simulink model "l2_pj_experiment"  (Simulink 7.1)
settings: Solver=ode45  StartTime=0.0  StopTime=100  MaxStep=.1  RelTol=1e-3
model workspace (MAT data in the model file):
  b : Simulink.Parameter (value not decoded)
  Ts : Simulink.Parameter (value not decoded)
  plant_index : Simulink.Parameter (value not decoded)
  omega_traj : Simulink.Parameter (value not decoded)
  alpha : Simulink.Parameter (value not decoded)
  N : Simulink.Parameter (value not decoded)
  epsilon : Simulink.Parameter (value not decoded)
  kp : Simulink.Parameter (value not decoded)
  wp : Simulink.Parameter (value not decoded)
libraries: passive_control x9, simulink x5
settings Model: Creator=Administrator  LastModifiedBy=Administrator

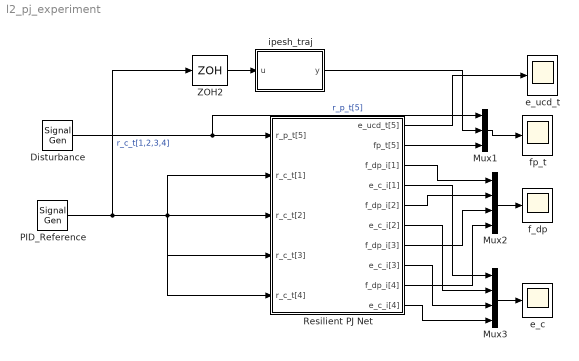
== system l2_pj_experiment ==
  Disturbance : SignalGenerator  WaveForm=square  Amplitude=.5  Frequency=.025
  Mux1 : Mux  Inputs=3
  Mux2 : Mux
  Mux3 : Mux
  PID_Reference : SignalGenerator  WaveForm=square  Frequency=.0125
  Resilient PJ Net : Subsystem
  ZOH2 : ZeroOrderHold  SampleTime=Ts
  e_c : Scope
      settings: SaveName=ScopeData2  SampleInput=on  SampleTime=Ts/10
  e_ucd_t : Scope
      settings: YMin=-1.1  YMax=1.1  SaveName=ScopeData3  SampleInput=on  SampleTime=Ts/10
  f_dp : Scope
      settings: TimeRange=100  SampleInput=on  SampleTime=Ts/10
  fp_t : Scope
      settings: TimeRange=100  YMin=-1.25  YMax=1.25  SampleInput=on  SampleTime=Ts/10
  ipesh_traj : Subsystem  mask{num=[omega_traj^2], den=[1,2*.9*omega_traj,omega_traj^2], Ts=Ts}
      mask prompts: num "H(s) num"; den "H(s) den"; Ts "Ts (sec)"
      mask init:
      | Hs=tf(num,den);
      | Hz=ipesh_transform(Hs,Ts);
  wires:
  PID_Reference/1 -> Resilient PJ Net/2(r_c_t[1]), Resilient PJ Net/3(r_c_t[2]), Resilient PJ Net/4(r_c_t[3]), Resilient PJ Net/5(r_c_t[4]), ZOH2/1  "r_c_t[1,2,3,4]"
  Disturbance/1 -> Resilient PJ Net/1(r_p_t[5]), Mux1/1  "r_p_t[5]"
  Mux2/1 -> f_dp/1
  Mux3/1 -> e_c/1
  Resilient PJ Net/1(e_ucd_t[5]) -> e_ucd_t/1
  Resilient PJ Net/10(e_c_i[4]) -> Mux3/4
  Resilient PJ Net/8(e_c_i[3]) -> Mux3/3
  Resilient PJ Net/6(e_c_i[2]) -> Mux3/2
  Resilient PJ Net/4(e_c_i[1]) -> Mux3/1
  Resilient PJ Net/3(f_dp_i[1]) -> Mux2/1
  Resilient PJ Net/5(f_dp_i[2]) -> Mux2/2
  Resilient PJ Net/7(f_dp_i[3]) -> Mux2/3
  Resilient PJ Net/9(f_dp_i[4]) -> Mux2/4
  Mux1/1 -> fp_t/1
  Resilient PJ Net/2(fp_t[5]) -> Mux1/3
  ZOH2/1 -> ipesh_traj/1(u)
  ipesh_traj/1(y) -> Mux1/2

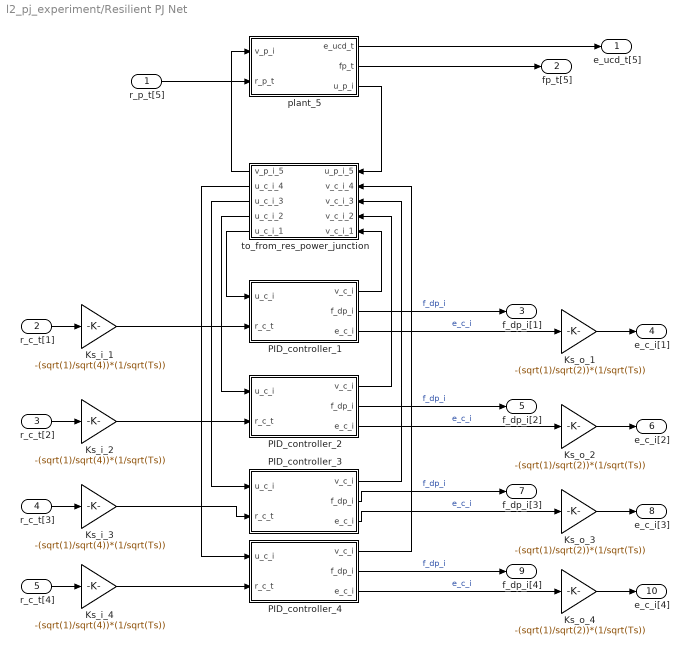
== system l2_pj_experiment/Resilient PJ Net ==
  r_p_t[5] : Inport
  r_c_t[1] : Inport  Port=2
  r_c_t[2] : Inport  Port=3
  r_c_t[3] : Inport  Port=4
  r_c_t[4] : Inport  Port=5
  Ks_i_{1..4} (4 alike) : Gain  Gain=-(sqrt(1)/sqrt(4))*(1/sqrt(Ts))  ParameterDataType=sfix(16)  ParameterScaling=2^0  OutDataType=sfix(16)  OutScaling=2^0
  Ks_o_{1..4} (4 alike) : Gain  Gain=-(sqrt(1)/sqrt(2))*(1/sqrt(Ts))  ParameterDataType=sfix(16)  ParameterScaling=2^0  OutDataType=sfix(16)  OutScaling=2^0
  PID_controller_1 : Subsystem
  PID_controller_2 : Subsystem
  PID_controller_3 : Subsystem
  PID_controller_4 : Subsystem
  plant_5 : Subsystem
  to_from_res_power_junction : Subsystem  Orientation=left
  e_ucd_t[5] : Outport
  fp_t[5] : Outport  Port=2
  f_dp_i[1] : Outport  Port=3
  e_c_i[1] : Outport  Port=4
  f_dp_i[2] : Outport  Port=5
  e_c_i[2] : Outport  Port=6
  f_dp_i[3] : Outport  Port=7
  e_c_i[3] : Outport  Port=8
  f_dp_i[4] : Outport  Port=9
  e_c_i[4] : Outport  Port=10
  wires:
  Ks_i_1/1 -> PID_controller_1/2(r_c_t)
  r_p_t[5]/1 -> plant_5/2(r_p_t)
  PID_controller_1/2(f_dp_i) -> f_dp_i[1]/1  "f_dp_i"
  r_c_t[1]/1 -> Ks_i_1/1
  PID_controller_1/3(e_c_i) -> Ks_o_1/1  "e_c_i"
  Ks_o_1/1 -> e_c_i[1]/1
  plant_5/1(e_ucd_t) -> e_ucd_t[5]/1
  plant_5/2(fp_t) -> fp_t[5]/1
  plant_5/3(u_p_i) -> to_from_res_power_junction/1(u_p_i_5)
  to_from_res_power_junction/1(v_p_i_5) -> plant_5/1(v_p_i)
  PID_controller_1/1(v_c_i) -> to_from_res_power_junction/5(v_c_i_1)
  to_from_res_power_junction/5(u_c_i_1) -> PID_controller_1/1(u_c_i)
  Ks_i_2/1 -> PID_controller_2/2(r_c_t)
  PID_controller_2/2(f_dp_i) -> f_dp_i[2]/1  "f_dp_i"
  r_c_t[2]/1 -> Ks_i_2/1
  PID_controller_2/3(e_c_i) -> Ks_o_2/1  "e_c_i"
  Ks_o_2/1 -> e_c_i[2]/1
  Ks_i_3/1 -> PID_controller_3/2(r_c_t)
  PID_controller_3/2(f_dp_i) -> f_dp_i[3]/1  "f_dp_i"
  r_c_t[3]/1 -> Ks_i_3/1
  PID_controller_3/3(e_c_i) -> Ks_o_3/1  "e_c_i"
  Ks_o_3/1 -> e_c_i[3]/1
  Ks_i_4/1 -> PID_controller_4/2(r_c_t)
  PID_controller_4/2(f_dp_i) -> f_dp_i[4]/1  "f_dp_i"
  r_c_t[4]/1 -> Ks_i_4/1
  PID_controller_4/3(e_c_i) -> Ks_o_4/1  "e_c_i"
  Ks_o_4/1 -> e_c_i[4]/1
  PID_controller_2/1(v_c_i) -> to_from_res_power_junction/4(v_c_i_2)
  to_from_res_power_junction/4(u_c_i_2) -> PID_controller_2/1(u_c_i)
  PID_controller_3/1(v_c_i) -> to_from_res_power_junction/3(v_c_i_3)
  to_from_res_power_junction/3(u_c_i_3) -> PID_controller_3/1(u_c_i)
  PID_controller_4/1(v_c_i) -> to_from_res_power_junction/2(v_c_i_4)
  to_from_res_power_junction/2(u_c_i_4) -> PID_controller_4/1(u_c_i)

== system l2_pj_experiment/ipesh_traj ==
  u : Inport
  ipesh : DiscreteTransferFcn  Numerator=Hz.num{1}  Denominator=Hz.den{1}  SampleTime=-1
  y : Outport
  wires:
  u/1 -> ipesh/1
  ipesh/1 -> y/1

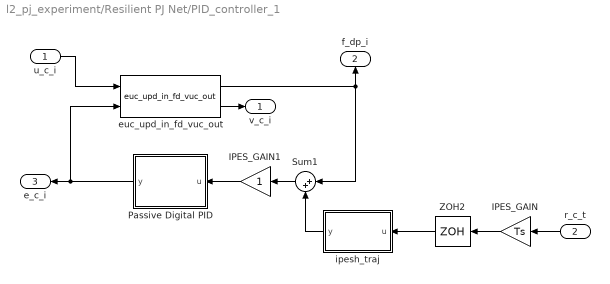
== system l2_pj_experiment/Resilient PJ Net/PID_controller_1 ==
  u_c_i : Inport
  r_c_t : Inport  Orientation=left  Port=2
  IPES_GAIN : Gain  Orientation=left  Gain=Ts  ParameterDataType=sfix(16)  ParameterScaling=2^0  OutDataType=sfix(16)  OutScaling=2^0
  IPES_GAIN1 : Gain  Orientation=left  ParameterDataType=sfix(16)  ParameterScaling=2^0  OutDataType=sfix(16)  OutScaling=2^0
  Passive Digital PID : Subsystem  Orientation=left  mask{kpk=kp, wpk=wp, alpha=alpha, N=N, Ts=Ts, epsilon=epsilon}
      mask prompts: kpk "Enter Plant Gains kpk (Vector)"; wpk "Enter Plant Frequencies wpk (Vector)"; alpha "Enter Alpha"; N "Enter N"; Ts "Sample Time [Ts] (seconds)"; epsilon "Enter epsiolon"
      mask init:
      | ksk=kpk./wpk;
      | kp=min(kpk);
      | wp=min(wpk);
      | wn=pi/Ts;
      | Kp=(1/3)*alpha*(wn+wp)/kp;
      | Ki=(1/3)*alpha*wn*(wn+wp)/kp;
      | Kd=(1/3)*alpha*(2/(N+1))*(wn+wp)/kp;
      | GIs=feedback(tf(Kp,[1,0]),epsilon);
      | GDs=Kd*tf([N*Ts/pi,1],[Ts/pi,1]);
  Sum1 : Sum  Orientation=left  Inputs=|++  OutDataType=sfix(16)  OutScaling=2^0
  ZOH2 : ZeroOrderHold  Orientation=left  SampleTime=Ts
  euc_upd_in_fd_vuc_out : passive_control/euc_upd_in_fd_vuc_out  SystemSampleTime=-1  b=b
  ipesh_traj : Subsystem  Orientation=left  mask{num=[omega_traj^2], den=[1,2*.9*omega_traj,omega_traj^2], Ts=Ts}
      mask prompts: num "H(s) num"; den "H(s) den"; Ts "Ts (sec)"
      mask init:
      | Hs=tf(num,den);
      | Hz=ipesh_transform(Hs,Ts);
  v_c_i : Outport
  f_dp_i : Outport  Orientation=up  Port=2
  e_c_i : Outport  Orientation=left  Port=3
  wires:
  euc_upd_in_fd_vuc_out/1 -> Sum1/1, f_dp_i/1
  ZOH2/1 -> ipesh_traj/1(u)
  r_c_t/1 -> IPES_GAIN/1
  Passive Digital PID/1(y) -> euc_upd_in_fd_vuc_out/2, e_c_i/1
  IPES_GAIN/1 -> ZOH2/1
  u_c_i/1 -> euc_upd_in_fd_vuc_out/1
  euc_upd_in_fd_vuc_out/2 -> v_c_i/1
  ipesh_traj/1(y) -> Sum1/2
  Sum1/1 -> IPES_GAIN1/1
  IPES_GAIN1/1 -> Passive Digital PID/1(u)

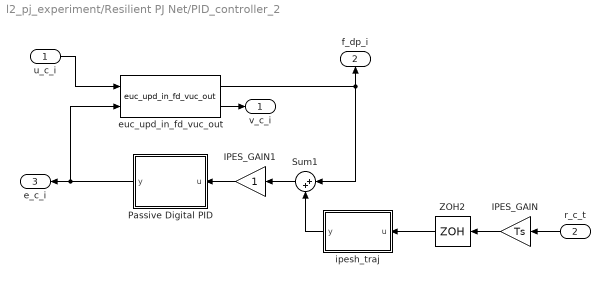
== system l2_pj_experiment/Resilient PJ Net/PID_controller_2 ==
  u_c_i : Inport
  r_c_t : Inport  Orientation=left  Port=2
  IPES_GAIN : Gain  Orientation=left  Gain=Ts  ParameterDataType=sfix(16)  ParameterScaling=2^0  OutDataType=sfix(16)  OutScaling=2^0
  IPES_GAIN1 : Gain  Orientation=left  ParameterDataType=sfix(16)  ParameterScaling=2^0  OutDataType=sfix(16)  OutScaling=2^0
  Passive Digital PID : Subsystem  Orientation=left  mask{kpk=kp, wpk=wp, alpha=alpha, N=N, Ts=Ts, epsilon=epsilon}
      mask prompts: kpk "Enter Plant Gains kpk (Vector)"; wpk "Enter Plant Frequencies wpk (Vector)"; alpha "Enter Alpha"; N "Enter N"; Ts "Sample Time [Ts] (seconds)"; epsilon "Enter epsiolon"
      mask init: same as l2_pj_experiment/Resilient PJ Net/PID_controller_1/Passive Digital PID
  Sum1 : Sum  Orientation=left  Inputs=|++  OutDataType=sfix(16)  OutScaling=2^0
  ZOH2 : ZeroOrderHold  Orientation=left  SampleTime=Ts
  euc_upd_in_fd_vuc_out : passive_control/euc_upd_in_fd_vuc_out  SystemSampleTime=-1  b=b
  ipesh_traj : Subsystem  Orientation=left  mask{num=[omega_traj^2], den=[1,2*.9*omega_traj,omega_traj^2], Ts=Ts}
      mask prompts: num "H(s) num"; den "H(s) den"; Ts "Ts (sec)"
      mask init:
      | Hs=tf(num,den);
      | Hz=ipesh_transform(Hs,Ts);
  v_c_i : Outport
  f_dp_i : Outport  Orientation=up  Port=2
  e_c_i : Outport  Orientation=left  Port=3
  wires:
  Sum1/1 -> IPES_GAIN1/1
  ipesh_traj/1(y) -> Sum1/2
  euc_upd_in_fd_vuc_out/2 -> v_c_i/1
  u_c_i/1 -> euc_upd_in_fd_vuc_out/1
  IPES_GAIN/1 -> ZOH2/1
  Passive Digital PID/1(y) -> e_c_i/1, euc_upd_in_fd_vuc_out/2
  r_c_t/1 -> IPES_GAIN/1
  ZOH2/1 -> ipesh_traj/1(u)
  euc_upd_in_fd_vuc_out/1 -> f_dp_i/1, Sum1/1
  IPES_GAIN1/1 -> Passive Digital PID/1(u)

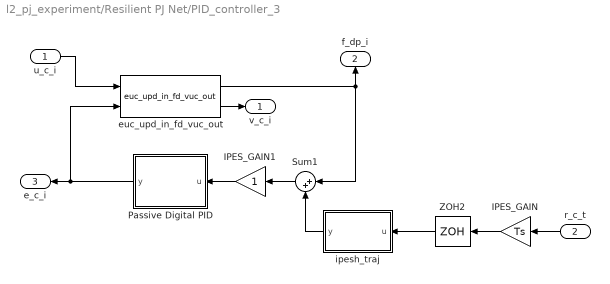
== system l2_pj_experiment/Resilient PJ Net/PID_controller_3 ==
  u_c_i : Inport
  r_c_t : Inport  Orientation=left  Port=2
  IPES_GAIN : Gain  Orientation=left  Gain=Ts  ParameterDataType=sfix(16)  ParameterScaling=2^0  OutDataType=sfix(16)  OutScaling=2^0
  IPES_GAIN1 : Gain  Orientation=left  ParameterDataType=sfix(16)  ParameterScaling=2^0  OutDataType=sfix(16)  OutScaling=2^0
  Passive Digital PID : Subsystem  Orientation=left  mask{kpk=kp, wpk=wp, alpha=alpha, N=N, Ts=Ts, epsilon=epsilon}
      mask prompts: kpk "Enter Plant Gains kpk (Vector)"; wpk "Enter Plant Frequencies wpk (Vector)"; alpha "Enter Alpha"; N "Enter N"; Ts "Sample Time [Ts] (seconds)"; epsilon "Enter epsiolon"
      mask init: same as l2_pj_experiment/Resilient PJ Net/PID_controller_1/Passive Digital PID
  Sum1 : Sum  Orientation=left  Inputs=|++  OutDataType=sfix(16)  OutScaling=2^0
  ZOH2 : ZeroOrderHold  Orientation=left  SampleTime=Ts
  euc_upd_in_fd_vuc_out : passive_control/euc_upd_in_fd_vuc_out  SystemSampleTime=-1  b=b
  ipesh_traj : Subsystem  Orientation=left  mask{num=[omega_traj^2], den=[1,2*.9*omega_traj,omega_traj^2], Ts=Ts}
      mask prompts: num "H(s) num"; den "H(s) den"; Ts "Ts (sec)"
      mask init:
      | Hs=tf(num,den);
      | Hz=ipesh_transform(Hs,Ts);
  v_c_i : Outport
  f_dp_i : Outport  Orientation=up  Port=2
  e_c_i : Outport  Orientation=left  Port=3
  wires:
  euc_upd_in_fd_vuc_out/1 -> Sum1/1, f_dp_i/1
  ZOH2/1 -> ipesh_traj/1(u)
  r_c_t/1 -> IPES_GAIN/1
  Passive Digital PID/1(y) -> euc_upd_in_fd_vuc_out/2, e_c_i/1
  IPES_GAIN/1 -> ZOH2/1
  u_c_i/1 -> euc_upd_in_fd_vuc_out/1
  euc_upd_in_fd_vuc_out/2 -> v_c_i/1
  ipesh_traj/1(y) -> Sum1/2
  Sum1/1 -> IPES_GAIN1/1
  IPES_GAIN1/1 -> Passive Digital PID/1(u)

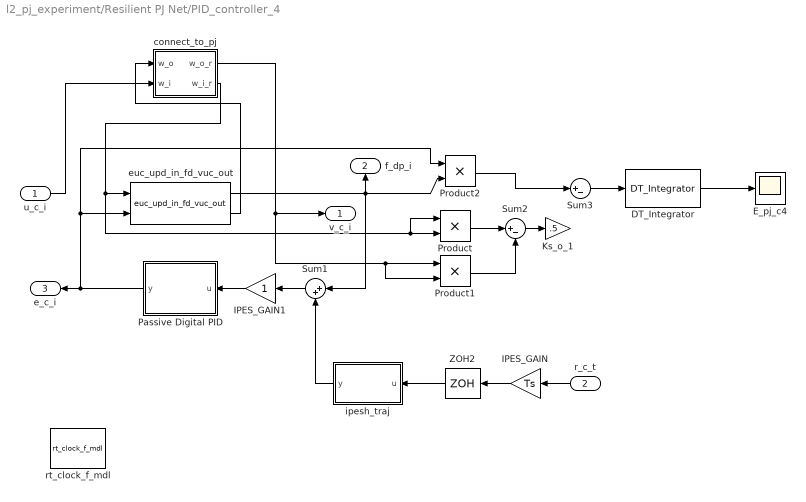
== system l2_pj_experiment/Resilient PJ Net/PID_controller_4 ==
  u_c_i : Inport
  r_c_t : Inport  Orientation=left  Port=2
  DT_Integrator : passive_control/passive_down_sampler/DT_Integrator  SystemSampleTime=-1
  E_pj_c4 : Scope
      settings: SaveName=ScopeData5
  IPES_GAIN : Gain  Orientation=left  Gain=Ts  ParameterDataType=sfix(16)  ParameterScaling=2^0  OutDataType=sfix(16)  OutScaling=2^0
  IPES_GAIN1 : Gain  Orientation=left  ParameterDataType=sfix(16)  ParameterScaling=2^0  OutDataType=sfix(16)  OutScaling=2^0
  Ks_o_1 : Gain  Gain=.5  ParameterDataType=sfix(16)  ParameterScaling=2^0  OutDataType=sfix(16)  OutScaling=2^0
  Passive Digital PID : Subsystem  Orientation=left  mask{kpk=kp, wpk=wp, alpha=alpha, N=N, Ts=Ts, epsilon=epsilon}
      mask prompts: kpk "Enter Plant Gains kpk (Vector)"; wpk "Enter Plant Frequencies wpk (Vector)"; alpha "Enter Alpha"; N "Enter N"; Ts "Sample Time [Ts] (seconds)"; epsilon "Enter epsiolon"
      mask init: same as l2_pj_experiment/Resilient PJ Net/PID_controller_1/Passive Digital PID
  Product : Product  OutDataType=sfix(16)  OutScaling=2^0  RndMeth=Zero
  Product1 : Product  OutDataType=sfix(16)  OutScaling=2^0  RndMeth=Zero
  Product2 : Product  OutDataType=sfix(16)  OutScaling=2^0  RndMeth=Zero
  Sum1 : Sum  Orientation=left  Inputs=|++  OutDataType=sfix(16)  OutScaling=2^0
  Sum2 : Sum  Inputs=|+-  OutDataType=sfix(16)  OutScaling=2^0
  Sum3 : Sum  Inputs=|+-  OutDataType=sfix(16)  OutScaling=2^0
  ZOH2 : ZeroOrderHold  Orientation=left  SampleTime=Ts
  connect_to_pj : Subsystem  mask{connect=on}
  euc_upd_in_fd_vuc_out : passive_control/euc_upd_in_fd_vuc_out  SystemSampleTime=-1  b=b
  ipesh_traj : Subsystem  Orientation=left  mask{num=[omega_traj^2], den=[1,2*.9*omega_traj,omega_traj^2], Ts=Ts}
      mask prompts: num "H(s) num"; den "H(s) den"; Ts "Ts (sec)"
      mask init:
      | Hs=tf(num,den);
      | Hz=ipesh_transform(Hs,Ts);
  rt_clock_f_mdl : passive_control/rt_clock_f_mdl  SystemSampleTime=-1  Ts=Ts  ID=1
  v_c_i : Outport
  f_dp_i : Outport  Orientation=up  Port=2
  e_c_i : Outport  Orientation=left  Port=3
  wires:
  Sum1/1 -> IPES_GAIN1/1
  ipesh_traj/1(y) -> Sum1/2
  IPES_GAIN/1 -> ZOH2/1
  Passive Digital PID/1(y) -> e_c_i/1, euc_upd_in_fd_vuc_out/2, Product2/1
  r_c_t/1 -> IPES_GAIN/1
  ZOH2/1 -> ipesh_traj/1(u)
  euc_upd_in_fd_vuc_out/1 -> f_dp_i/1, Product2/2, Sum1/1
  Product/1 -> Sum2/1
  Product1/1 -> Sum2/2
  Sum2/1 -> Ks_o_1/1
  Product2/1 -> Sum3/1
  Sum3/1 -> DT_Integrator/1
  DT_Integrator/1 -> E_pj_c4/1
  IPES_GAIN1/1 -> Passive Digital PID/1(u)
  u_c_i/1 -> connect_to_pj/2(w_i)
  connect_to_pj/2(w_i_r) -> euc_upd_in_fd_vuc_out/1, Product/2, Product/1
  euc_upd_in_fd_vuc_out/2 -> connect_to_pj/1(w_o)
  connect_to_pj/1(w_o_r) -> v_c_i/1, Product1/2, Product1/1

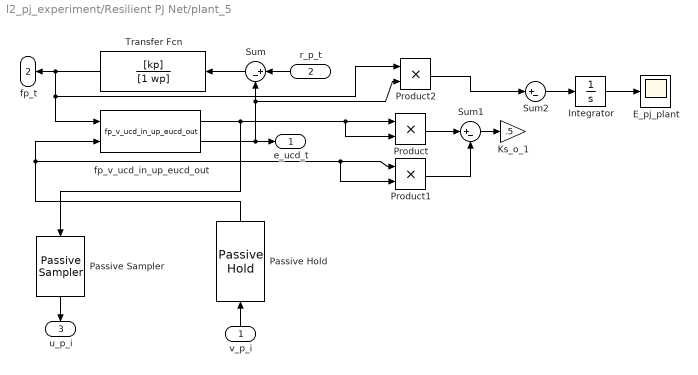
== system l2_pj_experiment/Resilient PJ Net/plant_5 ==
  v_p_i : Inport  Orientation=up
  r_p_t : Inport  Orientation=left  Port=2
  E_pj_plant : Scope
      settings: SaveName=ScopeData4  SampleInput=on  SampleTime=Ts
  Integrator : Integrator
  Ks_o_1 : Gain  Gain=.5  ParameterDataType=sfix(16)  ParameterScaling=2^0  OutDataType=sfix(16)  OutScaling=2^0
  Passive Hold : passive_control/Passive Hold  Orientation=up  SystemSampleTime=-1  Ts=Ts
  Passive Sampler : passive_control/Passive Sampler  Orientation=down  SystemSampleTime=-1  Ts=Ts
  Product : Product  OutDataType=sfix(16)  OutScaling=2^0  RndMeth=Zero
  Product1 : Product  OutDataType=sfix(16)  OutScaling=2^0  RndMeth=Zero
  Product2 : Product  OutDataType=sfix(16)  OutScaling=2^0  RndMeth=Zero
  Sum : Sum  Orientation=left  Inputs=|+-  OutDataType=sfix(16)  OutScaling=2^0
  Sum1 : Sum  Inputs=|+-  OutDataType=sfix(16)  OutScaling=2^0
  Sum2 : Sum  Inputs=|+-  OutDataType=sfix(16)  OutScaling=2^0
  Transfer Fcn : TransferFcn  Orientation=left  Numerator=[kp]  Denominator=[1 wp]
  fp_v_ucd_in_up_eucd_out : passive_control/fp_v_ucd_in_up_eucd_out  SystemSampleTime=-1  b=b
  e_ucd_t : Outport
  fp_t : Outport  Orientation=left  Port=2
  u_p_i : Outport  Orientation=down  Port=3
  wires:
  v_p_i/1 -> Passive Hold/1
  Passive Sampler/1 -> u_p_i/1
  Transfer Fcn/1 -> fp_t/1, fp_v_ucd_in_up_eucd_out/1, Product2/1
  Sum/1 -> Transfer Fcn/1
  r_p_t/1 -> Sum/1
  Passive Hold/1 -> fp_v_ucd_in_up_eucd_out/2, Product1/1, Product1/2
  fp_v_ucd_in_up_eucd_out/2 -> e_ucd_t/1, Sum/2, Product2/2
  fp_v_ucd_in_up_eucd_out/1 -> Passive Sampler/1, Product/1, Product/2
  Product/1 -> Sum1/1
  Product1/1 -> Sum1/2
  Sum1/1 -> Ks_o_1/1
  Product2/1 -> Sum2/1
  Sum2/1 -> Integrator/1
  Integrator/1 -> E_pj_plant/1

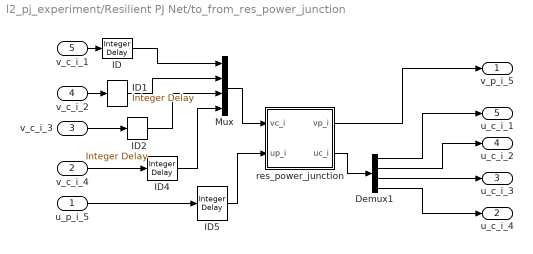
== system l2_pj_experiment/Resilient PJ Net/to_from_res_power_junction ==
  u_p_i_5 : Inport
  v_c_i_4 : Inport  Port=2
  v_c_i_3 : Inport  Port=3
  v_c_i_2 : Inport  Port=4
  v_c_i_1 : Inport  Port=5
  Demux1 : Demux
  ID{,1..2,4..5} (5 alike) : simulink/Discrete/Integer Delay  vinit=0.0  samptime=-1  NumDelays=2
  Mux : Mux
  res_power_junction : Subsystem  mask{ms=1, mc=4, Ts=Ts}
      mask prompts: ms "vector length [ms]"; mc "number of controllers [mc]"; Ts "sample rate (s) [Ts]"
  v_p_i_5 : Outport
  u_c_i_4 : Outport  Port=2
  u_c_i_3 : Outport  Port=3
  u_c_i_2 : Outport  Port=4
  u_c_i_1 : Outport  Port=5
  wires:
  Mux/1 -> res_power_junction/1(vc_i)
  u_p_i_5/1 -> ID5/1
  res_power_junction/2(uc_i) -> Demux1/1
  v_c_i_1/1 -> ID/1
  v_c_i_2/1 -> ID1/1
  v_c_i_3/1 -> ID2/1
  v_c_i_4/1 -> ID4/1
  res_power_junction/1(vp_i) -> v_p_i_5/1
  Demux1/1 -> u_c_i_1/1
  Demux1/2 -> u_c_i_2/1
  Demux1/3 -> u_c_i_3/1
  Demux1/4 -> u_c_i_4/1
  ID4/1 -> Mux/4
  ID5/1 -> res_power_junction/2(up_i)
  ID/1 -> Mux/1
  ID1/1 -> Mux/2
  ID2/1 -> Mux/3

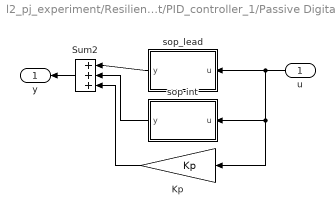
== system l2_pj_experiment/Resilient PJ Net/PID_controller_1/Passive Digital PID ==
  u : Inport  Orientation=left
  Kp : Gain  Orientation=left  Gain=Kp  ParameterDataType=sfix(16)  ParameterScaling=2^0  OutDataType=sfix(16)  OutScaling=2^0
  Sum2 : Sum  Orientation=left  Inputs=|+++  OutDataType=sfix(16)  OutScaling=2^0
  sop int : Subsystem  Orientation=left  mask{num=GIs.num{1}, den=GIs.den{1}, Ts=Ts}
      mask prompts: num "H(s) num"; den "H(s) den"; Ts "Ts (sec)"
      mask init:
      | Hs=tf(num,den);
      | Hz=ipesh_transform(Hs,Ts);
  sop_lead : Subsystem  Orientation=left  mask{num=GDs.num{1}, den=GDs.den{1}, Ts=Ts}
      mask prompts: num "H(s) num"; den "H(s) den"; Ts "Ts (sec)"
      mask init:
      | Hs=tf(num,den);
      | Hz=ipesh_transform(Hs,Ts);
  y : Outport  Orientation=left
  wires:
  u/1 -> sop_lead/1(u), Kp/1, sop int/1(u)
  sop_lead/1(y) -> Sum2/1
  sop int/1(y) -> Sum2/2
  Kp/1 -> Sum2/3
  Sum2/1 -> y/1

== system l2_pj_experiment/Resilient PJ Net/PID_controller_1/ipesh_traj ==
  u : Inport
  ipesh : DiscreteTransferFcn  Numerator=Hz.num{1}  Denominator=Hz.den{1}  SampleTime=-1
  y : Outport
  wires:
  ipesh/1 -> y/1
  u/1 -> ipesh/1

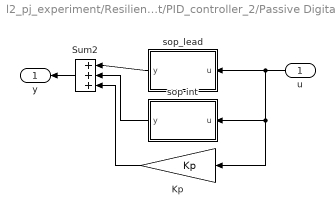
== system l2_pj_experiment/Resilient PJ Net/PID_controller_2/Passive Digital PID ==
  u : Inport  Orientation=left
  Kp : Gain  Orientation=left  Gain=Kp  ParameterDataType=sfix(16)  ParameterScaling=2^0  OutDataType=sfix(16)  OutScaling=2^0
  Sum2 : Sum  Orientation=left  Inputs=|+++  OutDataType=sfix(16)  OutScaling=2^0
  sop int : Subsystem  Orientation=left  mask{num=GIs.num{1}, den=GIs.den{1}, Ts=Ts}
      mask prompts: num "H(s) num"; den "H(s) den"; Ts "Ts (sec)"
      mask init:
      | Hs=tf(num,den);
      | Hz=ipesh_transform(Hs,Ts);
  sop_lead : Subsystem  Orientation=left  mask{num=GDs.num{1}, den=GDs.den{1}, Ts=Ts}
      mask prompts: num "H(s) num"; den "H(s) den"; Ts "Ts (sec)"
      mask init:
      | Hs=tf(num,den);
      | Hz=ipesh_transform(Hs,Ts);
  y : Outport  Orientation=left
  wires:
  Sum2/1 -> y/1
  Kp/1 -> Sum2/3
  sop int/1(y) -> Sum2/2
  sop_lead/1(y) -> Sum2/1
  u/1 -> sop int/1(u), Kp/1, sop_lead/1(u)

== system l2_pj_experiment/Resilient PJ Net/PID_controller_2/ipesh_traj ==
  u : Inport
  ipesh : DiscreteTransferFcn  Numerator=Hz.num{1}  Denominator=Hz.den{1}  SampleTime=-1
  y : Outport
  wires:
  u/1 -> ipesh/1
  ipesh/1 -> y/1

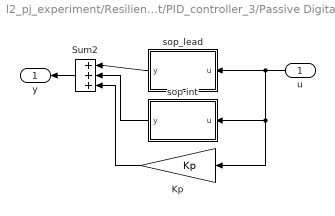
== system l2_pj_experiment/Resilient PJ Net/PID_controller_3/Passive Digital PID ==
  u : Inport  Orientation=left
  Kp : Gain  Orientation=left  Gain=Kp  ParameterDataType=sfix(16)  ParameterScaling=2^0  OutDataType=sfix(16)  OutScaling=2^0
  Sum2 : Sum  Orientation=left  Inputs=|+++  OutDataType=sfix(16)  OutScaling=2^0
  sop int : Subsystem  Orientation=left  mask{num=GIs.num{1}, den=GIs.den{1}, Ts=Ts}
      mask prompts: num "H(s) num"; den "H(s) den"; Ts "Ts (sec)"
      mask init:
      | Hs=tf(num,den);
      | Hz=ipesh_transform(Hs,Ts);
  sop_lead : Subsystem  Orientation=left  mask{num=GDs.num{1}, den=GDs.den{1}, Ts=Ts}
      mask prompts: num "H(s) num"; den "H(s) den"; Ts "Ts (sec)"
      mask init:
      | Hs=tf(num,den);
      | Hz=ipesh_transform(Hs,Ts);
  y : Outport  Orientation=left
  wires:
  u/1 -> sop_lead/1(u), Kp/1, sop int/1(u)
  sop_lead/1(y) -> Sum2/1
  sop int/1(y) -> Sum2/2
  Kp/1 -> Sum2/3
  Sum2/1 -> y/1

== system l2_pj_experiment/Resilient PJ Net/PID_controller_3/ipesh_traj ==
  u : Inport
  ipesh : DiscreteTransferFcn  Numerator=Hz.num{1}  Denominator=Hz.den{1}  SampleTime=-1
  y : Outport
  wires:
  ipesh/1 -> y/1
  u/1 -> ipesh/1

== system l2_pj_experiment/Resilient PJ Net/PID_controller_4/Passive Digital PID ==
  u : Inport  Orientation=left
  Kp : Gain  Orientation=left  Gain=Kp  ParameterDataType=sfix(16)  ParameterScaling=2^0  OutDataType=sfix(16)  OutScaling=2^0
  Sum2 : Sum  Orientation=left  Inputs=|+++  OutDataType=sfix(16)  OutScaling=2^0
  sop int : Subsystem  Orientation=left  mask{num=GIs.num{1}, den=GIs.den{1}, Ts=Ts}
      mask prompts: num "H(s) num"; den "H(s) den"; Ts "Ts (sec)"
      mask init:
      | Hs=tf(num,den);
      | Hz=ipesh_transform(Hs,Ts);
  sop_lead : Subsystem  Orientation=left  mask{num=GDs.num{1}, den=GDs.den{1}, Ts=Ts}
      mask prompts: num "H(s) num"; den "H(s) den"; Ts "Ts (sec)"
      mask init:
      | Hs=tf(num,den);
      | Hz=ipesh_transform(Hs,Ts);
  y : Outport  Orientation=left
  wires:
  Sum2/1 -> y/1
  Kp/1 -> Sum2/3
  sop int/1(y) -> Sum2/2
  sop_lead/1(y) -> Sum2/1
  u/1 -> sop_lead/1(u), Kp/1, sop int/1(u)

== system l2_pj_experiment/Resilient PJ Net/PID_controller_4/connect_to_pj ==
  w_o : Inport
  w_i : Inport  Port=2
  connect_to_pj : Stateflow chart
  w_o_r : Outport
  w_i_r : Outport  Port=2
  wires:
  connect_to_pj/2(w_i_r) -> w_i_r/1
  connect_to_pj/1(w_o_r) -> w_o_r/1
  w_i/1 -> connect_to_pj/2(w_i)
  w_o/1 -> connect_to_pj/1(w_o)

== system l2_pj_experiment/Resilient PJ Net/PID_controller_4/ipesh_traj ==
  u : Inport
  ipesh : DiscreteTransferFcn  Numerator=Hz.num{1}  Denominator=Hz.den{1}  SampleTime=-1
  y : Outport
  wires:
  u/1 -> ipesh/1
  ipesh/1 -> y/1

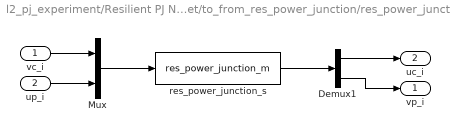
== system l2_pj_experiment/Resilient PJ Net/to_from_res_power_junction/res_power_junction ==
  vc_i : Inport
  up_i : Inport  Port=2
  Demux1 : Demux  Outputs=[4,1]
  Mux : Mux  Inputs=2
  res_power_junction_s : S-Function  FunctionName=res_power_junction_m  Parameters=ms,mc,Ts  EnableBusSupport=off
  vp_i : Outport
  uc_i : Outport  Port=2
  wires:
  vc_i/1 -> Mux/1
  up_i/1 -> Mux/2
  Demux1/1 -> uc_i/1
  Demux1/2 -> vp_i/1
  Mux/1 -> res_power_junction_s/1
  res_power_junction_s/1 -> Demux1/1

== system l2_pj_experiment/Resilient PJ Net/PID_controller_1/Passive Digital PID/sop int ==
  u : Inport
  ipesh : DiscreteTransferFcn  Numerator=Hz.num{1}  Denominator=Hz.den{1}  SampleTime=-1
  y : Outport
  wires:
  u/1 -> ipesh/1
  ipesh/1 -> y/1

== system l2_pj_experiment/Resilient PJ Net/PID_controller_1/Passive Digital PID/sop_lead ==
  u : Inport
  ipesh : DiscreteTransferFcn  Numerator=Hz.num{1}  Denominator=Hz.den{1}  SampleTime=-1
  y : Outport
  wires:
  u/1 -> ipesh/1
  ipesh/1 -> y/1

== system l2_pj_experiment/Resilient PJ Net/PID_controller_2/Passive Digital PID/sop int ==
  u : Inport
  ipesh : DiscreteTransferFcn  Numerator=Hz.num{1}  Denominator=Hz.den{1}  SampleTime=-1
  y : Outport
  wires:
  ipesh/1 -> y/1
  u/1 -> ipesh/1

== system l2_pj_experiment/Resilient PJ Net/PID_controller_2/Passive Digital PID/sop_lead ==
  u : Inport
  ipesh : DiscreteTransferFcn  Numerator=Hz.num{1}  Denominator=Hz.den{1}  SampleTime=-1
  y : Outport
  wires:
  ipesh/1 -> y/1
  u/1 -> ipesh/1

== system l2_pj_experiment/Resilient PJ Net/PID_controller_3/Passive Digital PID/sop int ==
  u : Inport
  ipesh : DiscreteTransferFcn  Numerator=Hz.num{1}  Denominator=Hz.den{1}  SampleTime=-1
  y : Outport
  wires:
  u/1 -> ipesh/1
  ipesh/1 -> y/1

== system l2_pj_experiment/Resilient PJ Net/PID_controller_3/Passive Digital PID/sop_lead ==
  u : Inport
  ipesh : DiscreteTransferFcn  Numerator=Hz.num{1}  Denominator=Hz.den{1}  SampleTime=-1
  y : Outport
  wires:
  u/1 -> ipesh/1
  ipesh/1 -> y/1

== system l2_pj_experiment/Resilient PJ Net/PID_controller_4/Passive Digital PID/sop int ==
  u : Inport
  ipesh : DiscreteTransferFcn  Numerator=Hz.num{1}  Denominator=Hz.den{1}  SampleTime=-1
  y : Outport
  wires:
  ipesh/1 -> y/1
  u/1 -> ipesh/1

== system l2_pj_experiment/Resilient PJ Net/PID_controller_4/Passive Digital PID/sop_lead ==
  u : Inport
  ipesh : DiscreteTransferFcn  Numerator=Hz.num{1}  Denominator=Hz.den{1}  SampleTime=-1
  y : Outport
  wires:
  ipesh/1 -> y/1
  u/1 -> ipesh/1

== matlab function Resilient PJ Net/PID_controller_4/connect_to_pj/connect_to_pj ==
  data: w_o input double; w_o_r output double; w_i input double; w_i_r output double; connect parameter double
function [w_o_r,w_i_r] = fcn(w_o, w_i, connect)
% This block supports the Embedded MATLAB subset.
% See the help menu for details. 
if connect
    w_o_r = w_o;
    w_i_r = w_i;
else
    w_o_r = 0*w_o;
    w_i_r = 0*w_i;
end
